simulink model "control_model_new_2018a_fuzzy"  (R2018a)
settings: Solver=VariableStepAuto  StartTime=0.0  StopTime=40  RelTol=1e-04
libraries: simulink x3, fuzblock x1
settings Model: Creator=geraldlow  LastModifiedBy=bcl15
settings DebuggingCC: LibraryContextMissingDiagnostic=warning
settings SFSimCC: SimUseLocalCustomCode=on
settings RTWCC: RTWUseLocalCustomCode=on

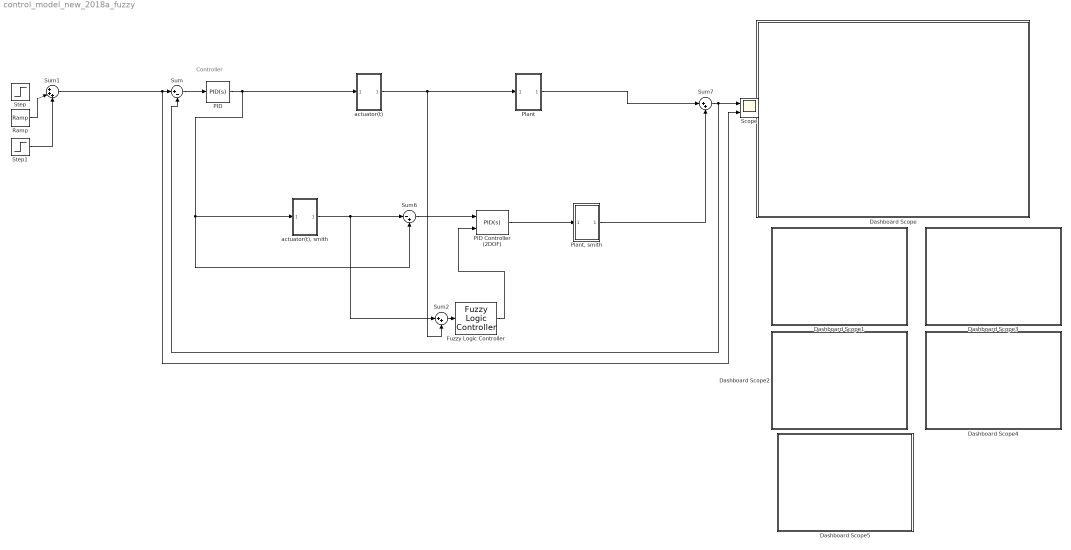
== system control_model_new_2018a_fuzzy ==
  note: Controller
  Dashboard Scope : Subsystem  DialogController=hmiCreateDDGDialog  IsWebBlock=on  mask(MWDashboardBlock){webBlockId=87415a21-a068-4dda-abbc-1e1ca7048776, webBlockType=sdiscope, ShowInLibBrowser=on, ShowInitialText=on, HMISrcModelName=control_model_new_2018a}
      mask prompts: webBlockId "WebBlock Id"; webBlockType "WebBlock Type"; HMISrcModelName "Source Model"
      mask help: Traces signals on the dashboard scope during simulation.
      mask Help: helpview([docroot '/mapfiles/simulink.map'], 'hmi_scope')
      mask Display:
      | if strcmp(get_param(bdroot(gcb),'BlockDiagramType'),'library')
      |  image([(matlabroot) '/toolbox/simulink/hmi/icons/SDIScope.png'])
      | end
  Dashboard Scope1 : Subsystem  DialogController=hmiCreateDDGDialog  IsWebBlock=on  mask(MWDashboardBlock){webBlockId=20a197ba-6778-4001-b82b-b1f8bd28131b, webBlockType=sdiscope, ShowInLibBrowser=on, ShowInitialText=on, HMISrcModelName=control_model_new_2018a}
      mask prompts: webBlockId "WebBlock Id"; webBlockType "WebBlock Type"; HMISrcModelName "Source Model"
      mask help: Traces signals on the dashboard scope during simulation.
      mask Help: helpview([docroot '/mapfiles/simulink.map'], 'hmi_scope')
      mask Display:
      | if strcmp(get_param(bdroot(gcb),'BlockDiagramType'),'library')
      |  image([(matlabroot) '/toolbox/simulink/hmi/icons/SDIScope.png'])
      | end
  Dashboard Scope2 : Subsystem  DialogController=hmiCreateDDGDialog  IsWebBlock=on  mask(MWDashboardBlock){webBlockId=a63d0e19-d6e7-4a8f-99b2-e0d4757ac662, webBlockType=sdiscope, ShowInLibBrowser=on, ShowInitialText=on, HMISrcModelName=control_model_new_2018a}
      mask prompts: webBlockId "WebBlock Id"; webBlockType "WebBlock Type"; HMISrcModelName "Source Model"
      mask help: Traces signals on the dashboard scope during simulation.
      mask Help: helpview([docroot '/mapfiles/simulink.map'], 'hmi_scope')
      mask Display:
      | if strcmp(get_param(bdroot(gcb),'BlockDiagramType'),'library')
      |  image([(matlabroot) '/toolbox/simulink/hmi/icons/SDIScope.png'])
      | end
  Dashboard Scope3 : Subsystem  DialogController=hmiCreateDDGDialog  IsWebBlock=on  mask(MWDashboardBlock){webBlockId=4e10b3f9-60b5-48cf-9052-a922590a3315, webBlockType=sdiscope, ShowInLibBrowser=on, ShowInitialText=on, HMISrcModelName=control_model_new_2018a}
      mask prompts: webBlockId "WebBlock Id"; webBlockType "WebBlock Type"; HMISrcModelName "Source Model"
      mask help: Traces signals on the dashboard scope during simulation.
      mask Help: helpview([docroot '/mapfiles/simulink.map'], 'hmi_scope')
      mask Display:
      | if strcmp(get_param(bdroot(gcb),'BlockDiagramType'),'library')
      |  image([(matlabroot) '/toolbox/simulink/hmi/icons/SDIScope.png'])
      | end
  Dashboard Scope4 : Subsystem  DialogController=hmiCreateDDGDialog  IsWebBlock=on  mask(MWDashboardBlock){webBlockId=bbff97e4-2399-4084-be8d-72d07d446755, webBlockType=sdiscope, ShowInitialText=on, HMISrcModelName=control_model_new_2018a}
      mask prompts: webBlockId "WebBlock Id"; webBlockType "WebBlock Type"; HMISrcModelName "Source Model"
      mask help: SimulinkHMI:dialogs:HMIScopeDialogDesc
      mask Help: helpview([docroot '/mapfiles/simulink.map'], 'hmi_scope')
      mask Display:
      | if strcmp(get_param(bdroot(gcb),'BlockDiagramType'), 'library')
      |     image([(matlabroot) '/toolbox/simulink/hmi/icons/DashboardScope.png']);
      | end
  Dashboard Scope5 : Subsystem  DialogController=hmiCreateDDGDialog  IsWebBlock=on  mask(MWDashboardBlock){webBlockId=e18ad3e5-8024-4d53-b240-27e72457439b, webBlockType=sdiscope, ShowInitialText=on, HMISrcModelName=control_model_new_2018a}
      mask prompts: webBlockId "WebBlock Id"; webBlockType "WebBlock Type"; HMISrcModelName "Source Model"
      mask help: SimulinkHMI:dialogs:HMIScopeDialogDesc
      mask Help: helpview([docroot '/mapfiles/simulink.map'], 'hmi_scope')
      mask Display:
      | if strcmp(get_param(bdroot(gcb),'BlockDiagramType'), 'library')
      |     image([(matlabroot) '/toolbox/simulink/hmi/icons/DashboardScope.png']);
      | end
  Fuzzy Logic Controller : fuzblock/Fuzzy Logic  Controller  FIS='tipper.fis'  OutputSampleNumber=101  DataType=double  FuzzifiedInputs=off  RuleFiringStrengths=off  RuleOutputs=off  AggregatedOutputs=off  SimulateUsing=Code generation  OutOfRangeInputValueMessage=warning  NoRuleFiredMessage=warning  EmptyOutputFuzzySetMessage=warning
  PID : simulink/Continuous/PID Controller  Controller=PID  TimeDomain=Continuous-time  SampleTime=-1  IntegratorMethod=Forward Euler  FilterMethod=Forward Euler  Form=Parallel  UseFilter=on  ControllerParametersSource=internal  P=135959466.906017  I=526081305890.553  D=6129.04665542498  N=108116.136818438  InitialConditionSource=internal  InitialConditionForIntegrator=0  InitialConditionForFilter=0  ExternalReset=none  LimitOutput=off  UpperSaturationLimit=inf  LowerSaturationLimit=-inf  LinearizeAsGain=on  AntiWindupMode=none  Kb=1  TrackingMode=off  Kt=1  PParamMin=[]  PParamMax=[]  IParamMin=[]  IParamMax=[]  DParamMin=[]  DParamMax=[]  NParamMin=[]  NParamMax=[]  KbParamMin=[]  KbParamMax=[]  KtParamMin=[]  KtParamMax=[]  POutMin=[]  POutMax=[]  IOutMin=[]  IOutMax=[]  DOutMin=[]  DOutMax=[]  NOutMin=[]  NOutMax=[]  KbOutMin=[]  KbOutMax=[]  KtOutMin=[]  KtOutMax=[]  IntegratorOutMin=[]  IntegratorOutMax=[]  FilterOutMin=[]  FilterOutMax=[]  SumOutMin=[]  SumOutMax=[]  SumI1OutMin=[]  SumI1OutMax=[]  SumI2OutMin=[]  SumI2OutMax=[]  SumI3OutMin=[]  SumI3OutMax=[]  SumDOutMin=[]  SumDOutMax=[]  SaturationOutMin=[]  SaturationOutMax=[]  IntegratorContinuousStateAttributes=''  IntegratorStateMustResolveToSignalObject=off  IntegratorRTWStateStorageClass=Auto  FilterContinuousStateAttributes=''  FilterStateMustResolveToSignalObject=off  FilterRTWStateStorageClass=Auto  DifferentiatorICPrevScaledInput=0  DifferentiatorOutMin=[]  DifferentiatorOutMax=[]  FilterDiffOutCoefMin=[]  FilterDiffOutCoefMax=[]  SumDenOutMin=[]  SumDenOutMax=[]  SumNumOutMin=[]  SumNumOutMax=[]  ReciprocalOutMin=[]  ReciprocalOutMax=[]  DivideOutMin=[]  DivideOutMax=[]  TunerSelectOption=Transfer Function Based (PID Tuner App)
  PID Controller (2DOF) : simulink/Continuous/PID Controller (2DOF)  Controller=PID  TimeDomain=Continuous-time  SampleTime=-1  IntegratorMethod=Forward Euler  FilterMethod=Forward Euler  Form=Parallel  UseFilter=on  ControllerParametersSource=internal  P=1  I=1  D=0  N=100  b=1  c=1  InitialConditionSource=internal  InitialConditionForIntegrator=0  InitialConditionForFilter=0  ExternalReset=none  LimitOutput=off  UpperSaturationLimit=inf  LowerSaturationLimit=-inf  LinearizeAsGain=on  AntiWindupMode=none  Kb=1  TrackingMode=off  Kt=1  PParamMin=[]  PParamMax=[]  IParamMin=[]  IParamMax=[]  DParamMin=[]  DParamMax=[]  NParamMin=[]  NParamMax=[]  bParamMin=[]  bParamMax=[]  cParamMin=[]  cParamMax=[]  KbParamMin=[]  KbParamMax=[]  KtParamMin=[]  KtParamMax=[]  POutMin=[]  POutMax=[]  IOutMin=[]  IOutMax=[]  DOutMin=[]  DOutMax=[]  NOutMin=[]  NOutMax=[]  bOutMin=[]  bOutMax=[]  cOutMin=[]  cOutMax=[]  KbOutMin=[]  KbOutMax=[]  KtOutMin=[]  KtOutMax=[]  IntegratorOutMin=[]  IntegratorOutMax=[]  FilterOutMin=[]  FilterOutMax=[]  SumOutMin=[]  SumOutMax=[]  Sum1OutMin=[]  Sum1OutMax=[]  Sum2OutMin=[]  Sum2OutMax=[]  Sum3OutMin=[]  Sum3OutMax=[]  SumI1OutMin=[]  SumI1OutMax=[]  SumI2OutMin=[]  SumI2OutMax=[]  SumI3OutMin=[]  SumI3OutMax=[]  SumDOutMin=[]  SumDOutMax=[]  SaturationOutMin=[]  SaturationOutMax=[]  IntegratorContinuousStateAttributes=''  IntegratorStateMustResolveToSignalObject=off  IntegratorRTWStateStorageClass=Auto  FilterContinuousStateAttributes=''  FilterStateMustResolveToSignalObject=off  FilterRTWStateStorageClass=Auto  DifferentiatorICPrevScaledInput=0  DifferentiatorOutMin=[]  DifferentiatorOutMax=[]  FilterDiffOutCoefMin=[]  FilterDiffOutCoefMax=[]  SumDenOutMin=[]  SumDenOutMax=[]  SumNumOutMin=[]  SumNumOutMax=[]  ReciprocalOutMin=[]  ReciprocalOutMax=[]  DivideOutMin=[]  DivideOutMax=[]  TunerSelectOption=Transfer Function Based (PID Tuner App)
  Plant : Subsystem
  "Plant, smith" : Subsystem
  Ramp : simulink/Sources/Ramp  slope=.125  start=15  InitialOutput=0
  Scope : Scope  NumInputPorts=2
  Step : Step  Time=10  After=.7  SampleTime=0
  Step1 : Step  Time=20  After=.5  SampleTime=0
  Sum : Sum  Inputs=|+-
  Sum1 : Sum  Inputs=|+++
  Sum2 : Sum  Inputs=|++
  Sum6 : Sum  Inputs=|-+
  Sum7 : Sum  Inputs=|++
  actuator(t) : Subsystem
  "actuator(t), smith" : Subsystem
  wires:
  Sum/1 -> PID/1
  Sum1/1 -> Sum/1, Scope/2
  Sum7/1 -> Sum/2, Scope/1
  PID/1 -> Sum6/2, "actuator(t), smith"/1(In1), actuator(t)/1(In1)
  Ramp/1 -> Sum1/2
  Step1/1 -> Sum1/3
  "actuator(t), smith"/1(Out1) -> Sum2/1, Sum6/1
  Plant/1(Out1) -> Sum7/1
  actuator(t)/1(Out1) -> Plant/1(In1), Sum2/2
  "Plant, smith"/1(Out1) -> Sum7/2
  Sum2/1 -> Fuzzy Logic Controller/1
  Fuzzy Logic Controller/1 -> PID Controller (2DOF)/2
  Sum6/1 -> PID Controller (2DOF)/1
  PID Controller (2DOF)/1 -> "Plant, smith"/1(In1)

== system control_model_new_2018a_fuzzy/Dashboard Scope ==

== system control_model_new_2018a_fuzzy/Dashboard Scope1 ==

== system control_model_new_2018a_fuzzy/Dashboard Scope2 ==

== system control_model_new_2018a_fuzzy/Dashboard Scope3 ==

== system control_model_new_2018a_fuzzy/Dashboard Scope4 ==

== system control_model_new_2018a_fuzzy/Dashboard Scope5 ==

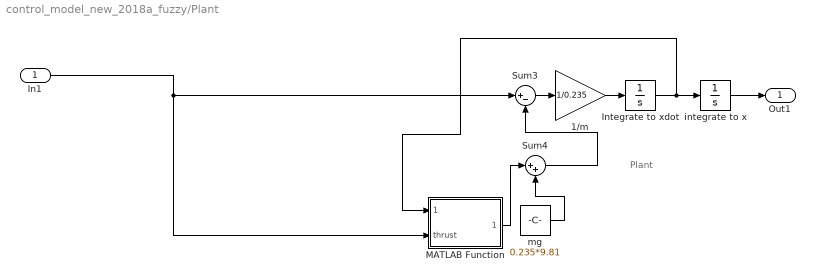
== system control_model_new_2018a_fuzzy/Plant ==
  note: Plant
  In1 : Inport
  1/m : Gain  Gain=1/0.235
  Integrate to xdot : Integrator
  MATLAB Function : MATLAB Function  TreatAsAtomicUnit=on
  Sum3 : Sum  Inputs=|+-
  Sum4 : Sum  Inputs=|++
  integrate to x : Integrator
  mg : Constant  Value=0.235*9.81
  Out1 : Outport
  wires:
  Integrate to xdot/1 -> MATLAB Function/1(velocity), integrate to x/1
  MATLAB Function/1(friction) -> Sum4/1
  1/m/1 -> Integrate to xdot/1
  Sum3/1 -> 1/m/1
  Sum4/1 -> Sum3/2
  In1/1 -> Sum3/1, MATLAB Function/2(thrust)
  mg/1 -> Sum4/2
  integrate to x/1 -> Out1/1

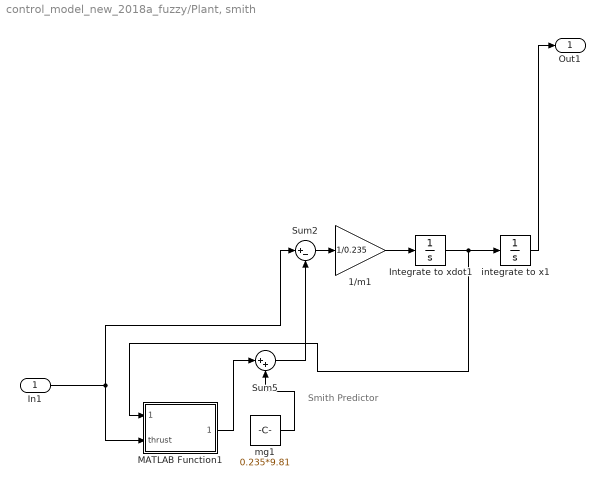
== system control_model_new_2018a_fuzzy/Plant, smith ==
  note: Smith Predictor
  In1 : Inport
  1/m1 : Gain  Gain=1/0.235
  Integrate to xdot1 : Integrator
  MATLAB Function1 : MATLAB Function  TreatAsAtomicUnit=on
  Sum2 : Sum  Inputs=|+-
  Sum5 : Sum  Inputs=|++
  integrate to x1 : Integrator
  mg1 : Constant  Value=0.235*9.81
  Out1 : Outport
  wires:
  Sum2/1 -> 1/m1/1
  Integrate to xdot1/1 -> integrate to x1/1, MATLAB Function1/1(velocity)
  Sum5/1 -> Sum2/2
  In1/1 -> MATLAB Function1/2(thrust), Sum2/1
  1/m1/1 -> Integrate to xdot1/1
  MATLAB Function1/1(friction) -> Sum5/1
  mg1/1 -> Sum5/2
  integrate to x1/1 -> Out1/1

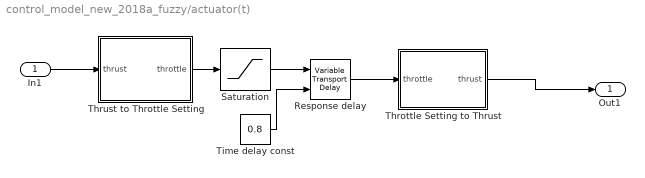
== system control_model_new_2018a_fuzzy/actuator(t) ==
  In1 : Inport
  Response delay : VariableTransportDelay  MaximumDelay=10
  Saturation : Saturate  UpperLimit=100  LowerLimit=0
  Throttle Setting to Thrust : MATLAB Function  TreatAsAtomicUnit=on
  Thrust to Throttle Setting : MATLAB Function  TreatAsAtomicUnit=on
  Time delay const : Constant  Value=0.8
  Out1 : Outport
  wires:
  Time delay const/1 -> Response delay/2
  Thrust to Throttle Setting/1(throttle) -> Saturation/1
  Response delay/1 -> Throttle Setting to Thrust/1(throttle)
  Throttle Setting to Thrust/1(thrust) -> Out1/1
  Saturation/1 -> Response delay/1
  In1/1 -> Thrust to Throttle Setting/1(thrust)

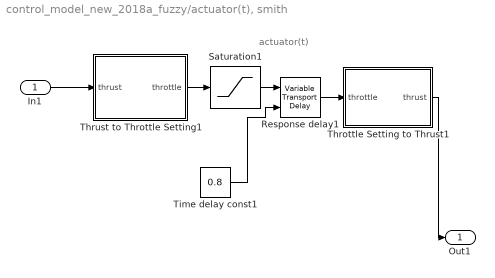
== system control_model_new_2018a_fuzzy/actuator(t), smith ==
  note: actuator(t)
  In1 : Inport
  Response delay1 : VariableTransportDelay  MaximumDelay=10
  Saturation1 : Saturate  UpperLimit=100  LowerLimit=0
  Throttle Setting to Thrust1 : MATLAB Function  TreatAsAtomicUnit=on
  Thrust to Throttle Setting1 : MATLAB Function  TreatAsAtomicUnit=on
  Time delay const1 : Constant  Value=0.8
  Out1 : Outport
  wires:
  Time delay const1/1 -> Response delay1/2
  Thrust to Throttle Setting1/1(throttle) -> Saturation1/1
  Response delay1/1 -> Throttle Setting to Thrust1/1(throttle)
  Saturation1/1 -> Response delay1/1
  Throttle Setting to Thrust1/1(thrust) -> Out1/1
  In1/1 -> Thrust to Throttle Setting1/1(thrust)

== matlab function control_model_new_2018a_fuzzy/actuator(t)/Throttle Setting to Thrust ==
  data: throttle input; thrust output
function thrust = fcn(throttle)
if throttle < 1
    thrust = 0;
elseif throttle > 88
    thrust=2*9.81*.66;
else
    thrust=2*9.81*(0.1+(.66-0.1)/(88-1)*(throttle-1));
end
end

== matlab function control_model_new_2018a_fuzzy/actuator(t)/Thrust to Throttle Setting ==
  data: thrust input; throttle output
function throttle = fcn(thrust)
% (.66-0.1)/(88-1)*2*9.81 = 0.1263
throttle = (thrust / 0.1263)+.8;
end

== matlab function control_model_new_2018a_fuzzy/Plant/MATLAB Function ==
  data: velocity input; friction output; thrust input
function friction   = fcn(velocity, thrust)
epsilon = 0.005; %small perturbation
mg = 0.235*9.81;
% Get reasonable values for x1, x2, l
x1 = 0.0125;
x2 = 0.0125;
l = 0.221;
netforce = thrust-mg; %mg should be a constant defined.
mu = 0.15; %coeff of dynamic friction
%static friction
if abs(velocity) < epsilon && abs(netforce) < 0.13*9.81 && netforce > 0
    friction = netforce;
elseif abs(velocity) < epsilon && abs(netforce) < 0.13*9.81 && netforce < 0
    friction = -netforce;
elseif velocity > 0
    friction=2*mu*(mg*x1-thrust*x2)/l;
elseif velocity < 0
    friction=-2*mu*(mg*x1-thrust*x2)/l;
else
    friction=0;
end

== matlab function control_model_new_2018a_fuzzy/Plant, smith/MATLAB Function1 ==
  data: velocity input; friction output; thrust input
function friction   = fcn(velocity, thrust)
epsilon = 0.005; %small perturbation
mg = 0.235*9.81;
% Get reasonable values for x1, x2, l
x1 = 0.0125;
x2 = 0.0125;
l = 0.221;
netforce = thrust-mg; %mg should be a constant defined.
mu = 0.15; %coeff of dynamic friction
%static friction
if abs(velocity) < epsilon && abs(netforce) < 0.13*9.81 && netforce > 0
    friction = netforce;
elseif abs(velocity) < epsilon && abs(netforce) < 0.13*9.81 && netforce < 0
    friction = -netforce;
elseif velocity > 0
    friction=2*mu*(mg*x1-thrust*x2)/l;
elseif velocity < 0
    friction=-2*mu*(mg*x1-thrust*x2)/l;
else
    friction=0;
end

== matlab function control_model_new_2018a_fuzzy/actuator(t), smith/Throttle Setting to Thrust1 ==
  data: throttle input; thrust output
function thrust = fcn(throttle)
if throttle < 1
    thrust = 0;
elseif throttle > 88
    thrust=2*9.81*.66;
else
    thrust=2*9.81*(0.1+(.66-0.1)/(88-1)*(throttle-1));
end
end

== matlab function control_model_new_2018a_fuzzy/actuator(t), smith/Thrust to Throttle Setting1 ==
  data: thrust input; throttle output
function throttle = fcn(thrust)
% (.66-0.1)/(88-1)*2*9.81 = 0.1263
throttle = (thrust / 0.1263)+.8;
end
